simulink model "HIL"  (R2022b)
settings: Solver=VariableStepAuto  StartTime=0.0  StopTime=60  RelTol=1e-3
undefined symbols (not defined in the file): LF
libraries: instrumentseriallib x3, etargetslib x1
settings Model: Creator=eic20nr  LastModifiedBy=nikil
settings ModelReferenceCC: EnableRefExpFcnMdlSchedulingChecks=on

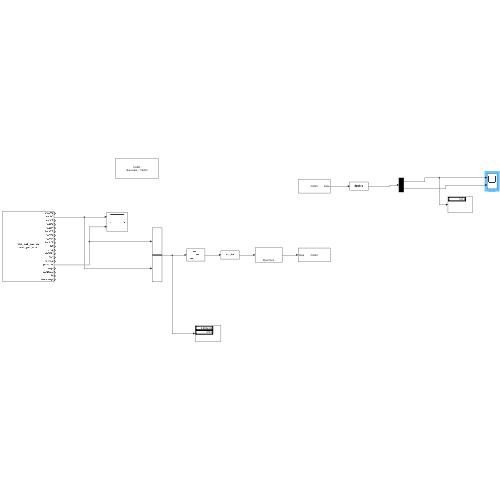
[thumbnail: Simulink's stored preview of the top-level diagram]
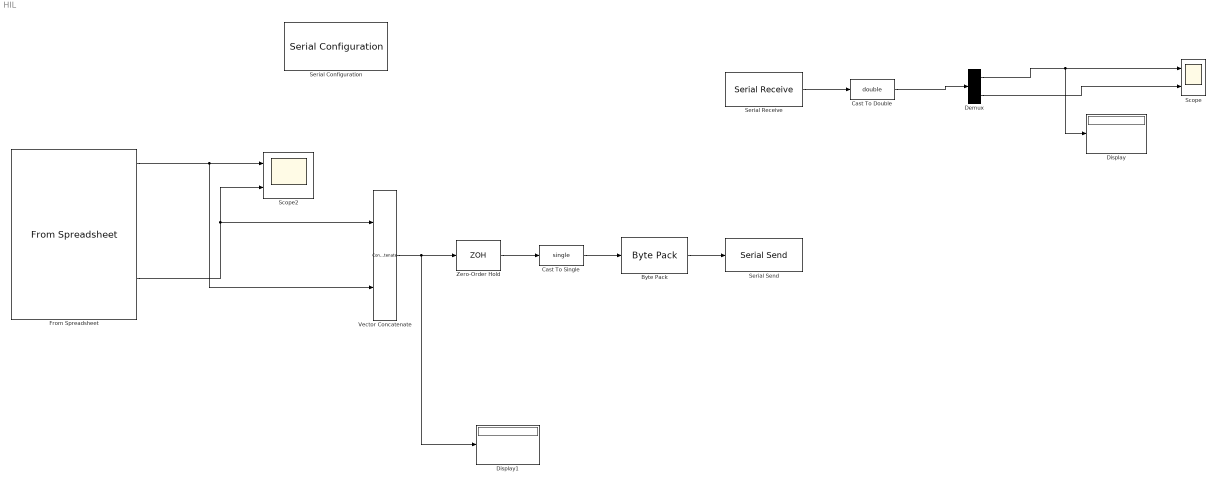
== system HIL ==
  Byte Pack : etargetslib/Byte Pack  datatypes={'single'}  byteAlign=4
  Cast To Double : DataTypeConversion  OutDataTypeStr=double  SaturateOnIntegerOverflow=off  RndMeth=Floor
  Cast To Single : DataTypeConversion  OutDataTypeStr=single  SaturateOnIntegerOverflow=off  RndMeth=Floor
  Demux : Demux  Outputs=2
  Display : Display
  Display1 : Display
  From Spreadsheet : FromSpreadsheet  FileName=more_pad_data.csv  SheetName=more_pad_data  SampleTime=0.05
  Scope : Scope  NumInputPorts=2
  Scope2 : Scope  NumInputPorts=2
  Serial Configuration : instrumentseriallib/Serial Configuration  Priority=-200000  PortSel=COM3  Port=COM3  ComPort=COM3  BaudRate=115200  DataBits=8  Parity=none  StopBits=1  ByteOrder=little-endian  FlowControl=none  Timeout=10  SimulateUsing=Interpreted execution  BlockInModel=on  aMode=1
  Serial Receive : instrumentseriallib/Serial Receive  Priority=1  PortSel=COM3  Port=COM3  ComPort=COM3  DataType=single  SaveDataType=uint8  ToggleHeader=on  Header='A'  ToggleTerminator=on  Terminator=LF ('\n')  CustomTerminator=[]  InputFormat=Column major  ToggleDataSize=on  DataSize=[1 2]  EnableBlockingMode=on  ActionDataUnavailable=Output last received value  ActionWhenDataUnavailable=Output last received value  CustomValue=0  SampleTime=0.05  SimulateUsing=Interpreted execution  BlockInModel=on  aMode=1
  Serial Send : instrumentseriallib/Serial Send  Priority=1  PortSel=COM3  Port=COM3  ComPort=COM3  Header=[]  Terminator=<none>  CustomTerminator=[]  EnableBlockingMode=on  SimulateUsing=Interpreted execution  BlockInModel=on  aMode=1
  Vector Concatenate : Concatenate
  Zero-Order Hold : ZeroOrderHold  SampleTime=0.05
  wires:
  Serial Receive/1 -> Cast To Double/1
  Cast To Double/1 -> Demux/1
  Zero-Order Hold/1 -> Cast To Single/1
  Cast To Single/1 -> Byte Pack/1
  Byte Pack/1 -> Serial Send/1
  Vector Concatenate/1 -> Zero-Order Hold/1, Display1/1
  Demux/1 -> Display/1, Scope/1
  Demux/2 -> Scope/2
  From Spreadsheet/2 -> Vector Concatenate/2, Scope2/1
  From Spreadsheet/15 -> Vector Concatenate/1, Scope2/2
